simulink model "roll_attitude"  (R2017a)
settings: Solver=VariableStepAuto  StartTime=0.0  StopTime=10.0  RelTol=1e-3
values from neighbouring files (symbols this model uses):
  a_phi1 = -P.rho*Va*P.S_wing*P.b^2*P.C_p_p/4    [computeRollGains.m]    (also in compute_gains.m)
  a_phi2 = P.rho*Va^2*P.S_wing*P.b*P.C_p_delta_a/2    [computeRollGains.m]    (also in compute_gains.m)
  delta_a_max = pi/4    (= 0.785398163397)    [computeRollGains.m]    (also in compute_gains.m)
  P = struct    [vehicle_params.m]
settings Model: Creator=pizzaslayer  LastModifiedBy=pizzaslayer

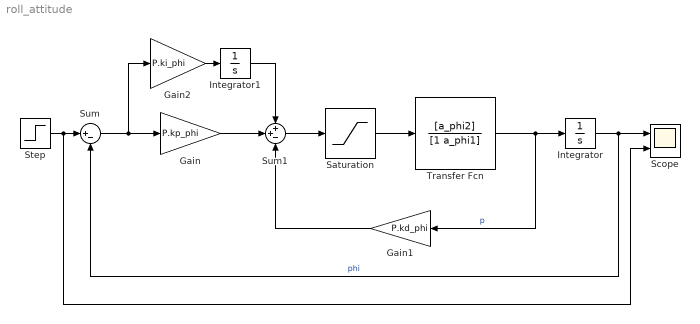
== system roll_attitude ==
  Gain : Gain  Gain=P.kp_phi
  Gain1 : Gain  Gain=P.kd_phi
  Gain2 : Gain  Gain=P.ki_phi
  Integrator : Integrator
  Integrator1 : Integrator
  Saturation : Saturate  UpperLimit=delta_a_max  LowerLimit=-delta_a_max
  Scope : Scope  NumInputPorts=2
  Step : Step  Time=0  SampleTime=0
  Sum : Sum  Inputs=|+-
  Sum1 : Sum  Inputs=++-
  Transfer Fcn : TransferFcn  Numerator=[a_phi2]  Denominator=[1 a_phi1]
  wires:
  Transfer Fcn/1 -> Gain1/1, Integrator/1  "p"
  Integrator/1 -> Sum/2, Scope/1  "phi"
  Step/1 -> Scope/2, Sum/1
  Sum/1 -> Gain2/1, Gain/1
  Gain/1 -> Sum1/2
  Gain1/1 -> Sum1/3
  Gain2/1 -> Integrator1/1
  Integrator1/1 -> Sum1/1
  Saturation/1 -> Transfer Fcn/1
  Sum1/1 -> Saturation/1
